simulink model "YXPChFPID"  (Simulink 7.8)
settings: Solver=ode45  SolverMode=SingleTasking  StartTime=0.0  StopTime=1  FixedStep=0.001  RelTol=1e-3
settings Model: Creator=Zhu Supeng  LastModifiedBy=Zhu Supeng
settings DataIOCC: SignalLoggingName=sigsOut
settings DebuggingCC: SaveWithParameterizedLinksMsg=none  SignalResolutionControl=TryResolveAllWithWarning  SolverPrmCheckMsg=none  MultiTaskDSMMsg=warning  MultiTaskCondExecSysMsg=none  StrictBusMsg=None
settings HardwareCC: TargetUnknown=on
settings RTWCC: IncludeERTFirstTime=on

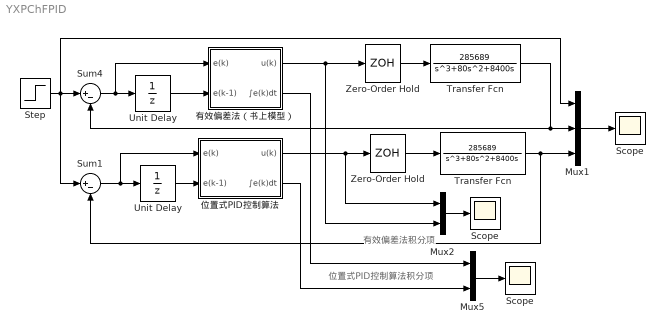
== system YXPChFPID ==
  note: 有效偏差法积分项
  note: 位置式PID控制算法积分项
  " Scope " : Scope
      settings: YMin=0  YMax=1.8  SaveName=YXPChFPIDI  DataFormat=Array  MaxDataPoints=500000
  Mux1 : Mux  Inputs=3
  Mux2 : Mux  Inputs=2
  Mux5 : Mux  Inputs=2
  Scope : Scope
      settings: YMin=30  YMax=34  SaveName=YXPChFPIDy  DataFormat=Array  MaxDataPoints=500000
  "Scope " : Scope
      settings: YMin=-3  YMax=6  SaveName=YXPChFPIDu  DataFormat=Array  MaxDataPoints=500000
  Step : Step  Time=0  After=30  SampleTime=0
  Sum1 : Sum  Inputs=|+-  SaturateOnIntegerOverflow=on
  Sum4 : Sum  Inputs=|+-  SaturateOnIntegerOverflow=on
  Transfer Fcn : TransferFcn  Numerator=[285689]  Denominator=[1 80 8400 0]
  "Transfer Fcn " : TransferFcn  Numerator=[285689]  Denominator=[1 80 8400 0]
  Unit Delay : UnitDelay  SampleTime=0.001
  "Unit Delay " : UnitDelay  SampleTime=0.001
  Zero-Order Hold : ZeroOrderHold  SampleTime=0.001
  "Zero-Order Hold " : ZeroOrderHold  SampleTime=0.001
  "位置式PID控制算法 " : Subsystem
  有效偏差法（书上模型） : Subsystem
  wires:
  Step/1 -> Sum4/1, Mux1/1, Sum1/1
  "位置式PID控制算法 "/1(u(k)) -> "Zero-Order Hold "/1, Mux2/1
  "Zero-Order Hold "/1 -> "Transfer Fcn "/1
  "Transfer Fcn "/1 -> Sum1/2, Mux1/3
  "Unit Delay "/1 -> "位置式PID控制算法 "/2(e(k-1))
  Sum1/1 -> "位置式PID控制算法 "/1(e(k)), "Unit Delay "/1
  Mux1/1 -> Scope/1
  有效偏差法（书上模型）/1(u(k)) -> Zero-Order Hold/1, Mux2/2
  Zero-Order Hold/1 -> Transfer Fcn/1
  Transfer Fcn/1 -> Sum4/2, Mux1/2
  Unit Delay/1 -> 有效偏差法（书上模型）/2(e(k-1))
  Sum4/1 -> Unit Delay/1, 有效偏差法（书上模型）/1(e(k))
  Mux2/1 -> "Scope "/1
  Mux5/1 -> " Scope "/1
  "位置式PID控制算法 "/2(∫e(k)dt) -> Mux5/2
  有效偏差法（书上模型）/2(∫e(k)dt) -> Mux5/1

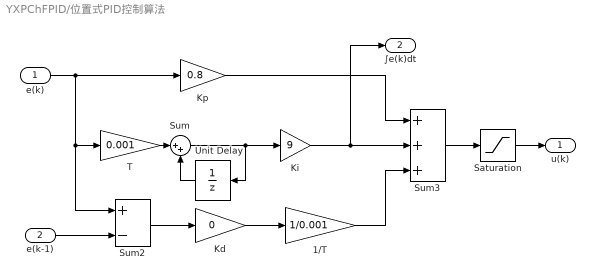
== system YXPChFPID/位置式PID控制算法  ==
  e(k) : Inport
  e(k-1) : Inport  Port=2
  1/T : Gain  Gain=1/0.001  SaturateOnIntegerOverflow=on  OutDataTypeStr=Inherit: Same as input  ParamDataTypeStr=Inherit: Same as input
  Kd : Gain  Gain=0  SaturateOnIntegerOverflow=on  OutDataTypeStr=Inherit: Same as input  ParamDataTypeStr=Inherit: Same as input
  Ki : Gain  Gain=9  SaturateOnIntegerOverflow=on  OutDataTypeStr=Inherit: Same as input  ParamDataTypeStr=Inherit: Same as input
  Kp : Gain  Gain=0.8  SaturateOnIntegerOverflow=on  OutDataTypeStr=Inherit: Same as input  ParamDataTypeStr=Inherit: Same as input
  Saturation : Saturate  UpperLimit=10  LowerLimit=-10
  Sum : Sum  Inputs=|++  SaturateOnIntegerOverflow=on
  Sum2 : Sum  Inputs=+-  SaturateOnIntegerOverflow=on
  Sum3 : Sum  Inputs=+++  SaturateOnIntegerOverflow=on
  T : Gain  Gain=0.001  SaturateOnIntegerOverflow=on  OutDataTypeStr=Inherit: Same as input  ParamDataTypeStr=Inherit: Same as input
  Unit Delay : UnitDelay  SampleTime=0.001
  u(k) : Outport
  ∫e(k)dt : Outport  Port=2
  wires:
  Ki/1 -> Sum3/2, ∫e(k)dt/1
  1/T/1 -> Sum3/3
  e(k-1)/1 -> Sum2/2
  Kd/1 -> 1/T/1
  Saturation/1 -> u(k)/1
  Sum3/1 -> Saturation/1
  Kp/1 -> Sum3/1
  e(k)/1 -> Kp/1, Sum2/1, T/1
  Sum2/1 -> Kd/1
  Sum/1 -> Unit Delay/1, Ki/1
  Unit Delay/1 -> Sum/2
  T/1 -> Sum/1

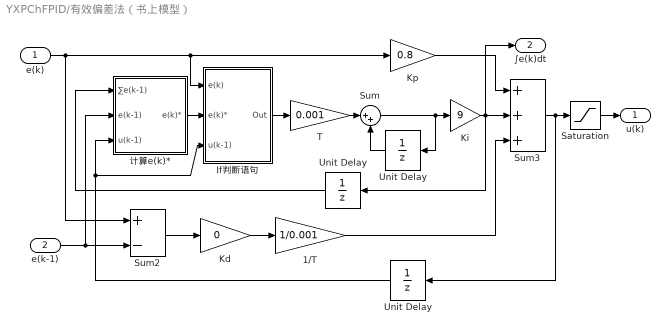
== system YXPChFPID/有效偏差法（书上模型） ==
  e(k) : Inport
  e(k-1) : Inport  Port=2
  " Unit Delay " : UnitDelay  SampleTime=0.001
  1/T : Gain  Gain=1/0.001  SaturateOnIntegerOverflow=on  OutDataTypeStr=Inherit: Same as input  ParamDataTypeStr=Inherit: Same as input
  If判断语句 : Subsystem
  Kd : Gain  Gain=0  SaturateOnIntegerOverflow=on  OutDataTypeStr=Inherit: Same as input  ParamDataTypeStr=Inherit: Same as input
  Ki : Gain  Gain=9  SaturateOnIntegerOverflow=on  OutDataTypeStr=Inherit: Same as input  ParamDataTypeStr=Inherit: Same as input
  Kp : Gain  Gain=0.8  SaturateOnIntegerOverflow=on  OutDataTypeStr=Inherit: Same as input  ParamDataTypeStr=Inherit: Same as input
  Saturation : Saturate  UpperLimit=10  LowerLimit=-10
  Sum : Sum  Inputs=|++  SaturateOnIntegerOverflow=on
  Sum2 : Sum  Inputs=+-  SaturateOnIntegerOverflow=on
  Sum3 : Sum  Inputs=+++  SaturateOnIntegerOverflow=on
  T : Gain  Gain=0.001  SaturateOnIntegerOverflow=on  OutDataTypeStr=Inherit: Same as input  ParamDataTypeStr=Inherit: Same as input
  Unit Delay : UnitDelay  SampleTime=0.001
  "Unit Delay " : UnitDelay  SampleTime=0.001
  计算e(k)* : Subsystem
  u(k) : Outport
  ∫e(k)dt : Outport  Port=2
  wires:
  Saturation/1 -> u(k)/1
  Sum2/1 -> Kd/1
  e(k)/1 -> If判断语句/1(e(k)), Kp/1, Sum2/1
  Kp/1 -> Sum3/1
  Sum3/1 -> Saturation/1, "Unit Delay "/1
  Kd/1 -> 1/T/1
  e(k-1)/1 -> Sum2/2, 计算e(k)*/2(e(k-1))
  1/T/1 -> Sum3/3
  Ki/1 -> Sum3/2, " Unit Delay "/1, ∫e(k)dt/1
  计算e(k)*/1(e(k)*) -> If判断语句/2("e(k)* ")
  " Unit Delay "/1 -> 计算e(k)*/1(∑e(k-1))
  If判断语句/1("Out ") -> T/1
  Sum/1 -> Unit Delay/1, Ki/1
  Unit Delay/1 -> Sum/2
  T/1 -> Sum/1
  "Unit Delay "/1 -> 计算e(k)*/3(u(k-1)), If判断语句/3(u(k-1))

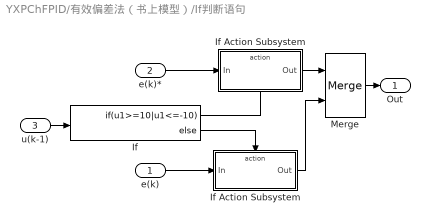
== system YXPChFPID/有效偏差法（书上模型）/If判断语句 ==
  e(k) : Inport
  "e(k)* " : Inport  Port=2
  u(k-1) : Inport  Port=3
  If : If  IfExpression=u1>=10|u1<=-10
  If Action Subsystem : Subsystem  TreatAsAtomicUnit=on
  "If Action Subsystem " : Subsystem  TreatAsAtomicUnit=on
  Merge : Merge
  "Out " : Outport
  wires:
  If/2 -> "If Action Subsystem "/Action
  e(k)/1 -> "If Action Subsystem "/1("In ")
  u(k-1)/1 -> If/1
  "If Action Subsystem "/1("Out ") -> Merge/2
  If Action Subsystem/1("Out ") -> Merge/1
  "e(k)* "/1 -> If Action Subsystem/1("In ")
  If/1 -> If Action Subsystem/Action
  Merge/1 -> "Out "/1

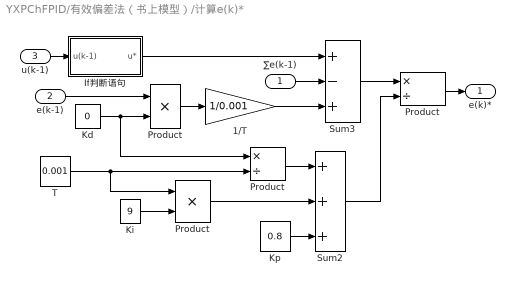
== system YXPChFPID/有效偏差法（书上模型）/计算e(k)* ==
  ∑e(k-1) : Inport
  e(k-1) : Inport  Port=2
  u(k-1) : Inport  Port=3
  " Product" : Product  SaturateOnIntegerOverflow=on  OutDataTypeStr=Inherit: Same as first input
  " Product " : Product  Inputs=*/  SaturateOnIntegerOverflow=on  OutDataTypeStr=Inherit: Same as first input
  1/T : Gain  Gain=1/0.001  SaturateOnIntegerOverflow=on  OutDataTypeStr=Inherit: Same as input  ParamDataTypeStr=Inherit: Same as input
  If判断语句 : Subsystem
  Kd : Constant  Value=0
  Ki : Constant  Value=9
  Kp : Constant  Value=0.8
  Product : Product  Inputs=*/  SaturateOnIntegerOverflow=on  OutDataTypeStr=Inherit: Same as first input
  "Product " : Product  SaturateOnIntegerOverflow=on  OutDataTypeStr=Inherit: Same as first input
  Sum2 : Sum  Inputs=+++  SaturateOnIntegerOverflow=on
  Sum3 : Sum  Inputs=+-+  SaturateOnIntegerOverflow=on
  T : Constant  Value=0.001
  e(k)* : Outport
  wires:
  Ki/1 -> " Product"/2
  "Product "/1 -> 1/T/1
  e(k-1)/1 -> "Product "/1
  1/T/1 -> Sum3/3
  Sum3/1 -> Product/1
  Kd/1 -> "Product "/2, " Product "/1
  T/1 -> " Product"/1, " Product "/2
  " Product "/1 -> Sum2/1
  " Product"/1 -> Sum2/2
  Kp/1 -> Sum2/3
  Sum2/1 -> Product/2
  Product/1 -> e(k)*/1
  u(k-1)/1 -> If判断语句/1(u(k-1))
  ∑e(k-1)/1 -> Sum3/2
  If判断语句/1("u* ") -> Sum3/1

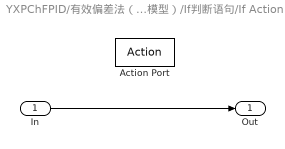
== system YXPChFPID/有效偏差法（书上模型）/If判断语句/If Action Subsystem ==
  "In " : Inport
  Action Port : ActionPort  ActionType=then
  "Out " : Outport
  wires:
  "In "/1 -> "Out "/1

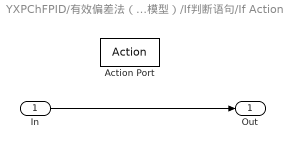
== system YXPChFPID/有效偏差法（书上模型）/If判断语句/If Action Subsystem  ==
  "In " : Inport
  Action Port : ActionPort  ActionType=else
  "Out " : Outport
  wires:
  "In "/1 -> "Out "/1

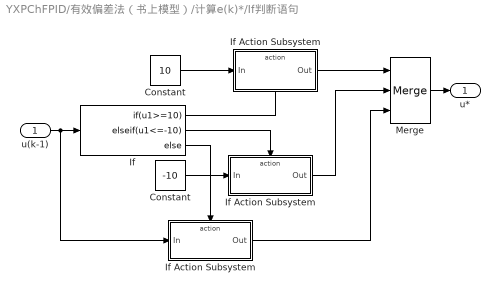
== system YXPChFPID/有效偏差法（书上模型）/计算e(k)*/If判断语句 ==
  u(k-1) : Inport
  Constant : Constant  Value=-10
  "Constant " : Constant  Value=10
  If : If  IfExpression=u1>=10  ElseIfExpressions=u1<=-10
  If Action Subsystem : Subsystem  TreatAsAtomicUnit=on
  "If Action Subsystem " : Subsystem  TreatAsAtomicUnit=on
  "If Action Subsystem  " : Subsystem  TreatAsAtomicUnit=on
  Merge : Merge  Inputs=3
  "u* " : Outport
  wires:
  Constant/1 -> "If Action Subsystem  "/1("In ")
  u(k-1)/1 -> If/1, "If Action Subsystem "/1("In ")
  "If Action Subsystem  "/1("Out ") -> Merge/2
  If Action Subsystem/1("Out ") -> Merge/1
  "Constant "/1 -> If Action Subsystem/1("In ")
  If/1 -> If Action Subsystem/Action
  Merge/1 -> "u* "/1
  If/2 -> "If Action Subsystem  "/Action
  If/3 -> "If Action Subsystem "/Action
  "If Action Subsystem "/1("Out ") -> Merge/3

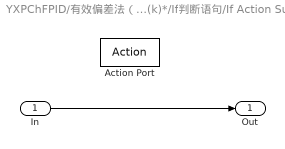
== system YXPChFPID/有效偏差法（书上模型）/计算e(k)*/If判断语句/If Action Subsystem ==
  "In " : Inport
  Action Port : ActionPort  ActionType=then
  "Out " : Outport
  wires:
  "In "/1 -> "Out "/1

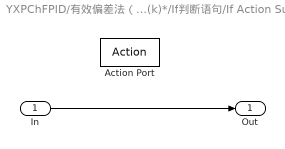
== system YXPChFPID/有效偏差法（书上模型）/计算e(k)*/If判断语句/If Action Subsystem  ==
  "In " : Inport
  Action Port : ActionPort  ActionType=else
  "Out " : Outport
  wires:
  "In "/1 -> "Out "/1

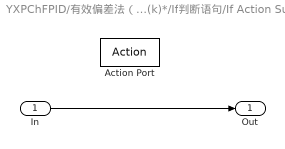
== system YXPChFPID/有效偏差法（书上模型）/计算e(k)*/If判断语句/If Action Subsystem   ==
  "In " : Inport
  Action Port : ActionPort  ActionType=elseif
  "Out " : Outport
  wires:
  "In "/1 -> "Out "/1
